simulink model "scalar_training_simulink"  (R2024a)
settings: Solver=FixedStepAuto  StartTime=0.0  StopTime=time(end)  FixedStep=ST  RelTol=1e-3
values from neighbouring files (symbols this model uses):
  c_init = (1/n_nodes)*ones(1, n_nodes)    [scalar_training_init.m]
  delta = 1.2*u_amplitude/(n_nodes/2)    (= 0.072)    [scalar_training_init.m]
  k_a = 0.1    [scalar_training_init.m]
  n_nodes = 50    [scalar_training_init.m]
  ST = 1    [scalar_training_init.m]
settings Model: Creator=gabri  LastModifiedBy=gabri

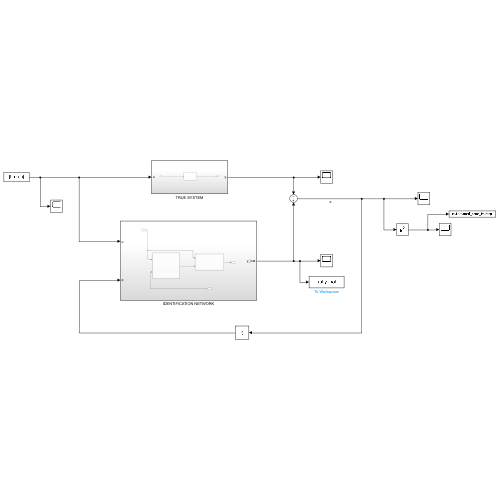
[thumbnail: Simulink's stored preview of the top-level diagram]
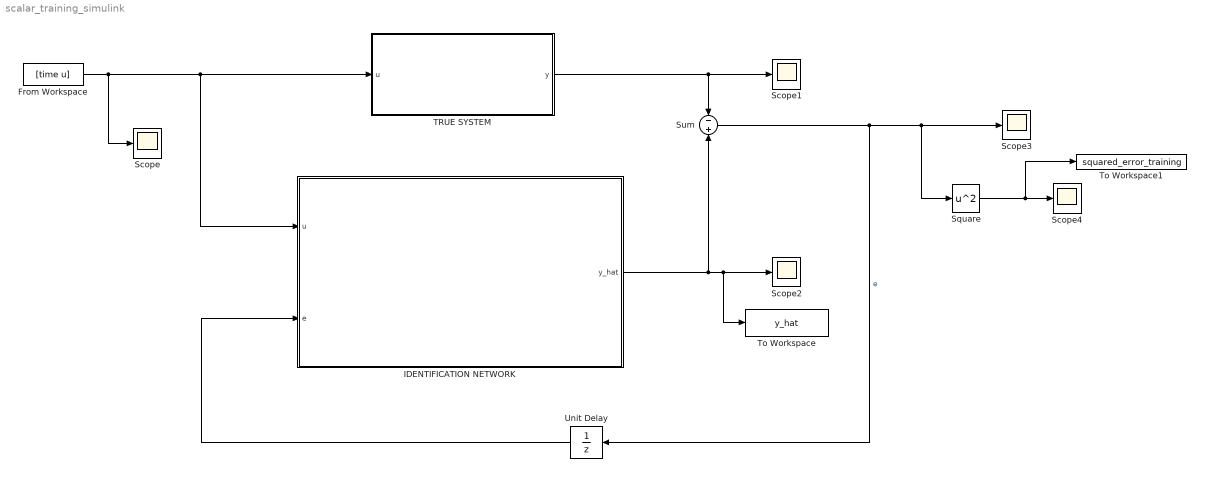
== system scalar_training_simulink ==
  From Workspace : FromWorkspace  VariableName=[time u]  SampleTime=ST
  IDENTIFICATION NETWORK : Subsystem
  Scope{,1..4} (5 alike) : Scope
  Square : Math  Operator=square
  Sum : Sum  Inputs=-|+
  TRUE SYSTEM : Subsystem
  To Workspace : ToWorkspace  VariableName=y_hat  SaveFormat=Timeseries  SampleTime=-1
  To Workspace1 : ToWorkspace  VariableName=squared_error_training  SaveFormat=Timeseries  SampleTime=-1
  Unit Delay : UnitDelay  SampleTime=ST  HasFrameUpgradeWarning=on
  wires:
  From Workspace/1 -> IDENTIFICATION NETWORK/1(u), TRUE SYSTEM/1(u), Scope/1
  TRUE SYSTEM/1(y) -> Sum/1, Scope1/1
  Sum/1 -> Scope3/1, Square/1, Unit Delay/1  "e"
  Square/1 -> To Workspace1/1, Scope4/1
  IDENTIFICATION NETWORK/1(y_hat) -> To Workspace/1, Scope2/1, Sum/2
  Unit Delay/1 -> IDENTIFICATION NETWORK/2(e)

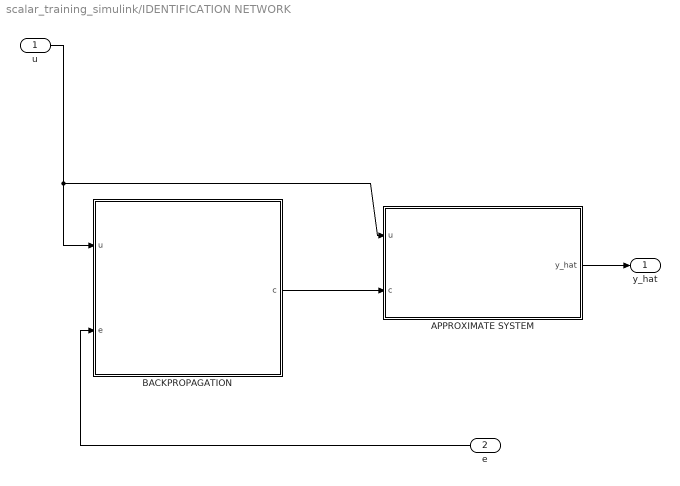
== system scalar_training_simulink/IDENTIFICATION NETWORK ==
  u : Inport
  e : Inport  Port=2
  APPROXIMATE SYSTEM : Subsystem
  BACKPROPAGATION : Subsystem
  y_hat : Outport
  wires:
  BACKPROPAGATION/1(c) -> APPROXIMATE SYSTEM/2(c)
  u/1 -> BACKPROPAGATION/1(u), APPROXIMATE SYSTEM/1(u)
  APPROXIMATE SYSTEM/1(y_hat) -> y_hat/1
  e/1 -> BACKPROPAGATION/2(e)

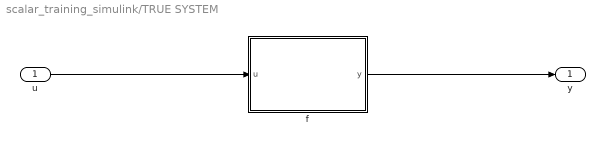
== system scalar_training_simulink/TRUE SYSTEM ==
  u : Inport
  f : MATLAB Function  TreatAsAtomicUnit=on
  y : Outport
  wires:
  u/1 -> f/1(u)
  f/1(y) -> y/1

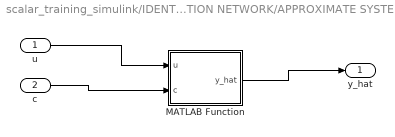
== system scalar_training_simulink/IDENTIFICATION NETWORK/APPROXIMATE SYSTEM ==
  u : Inport
  c : Inport  Port=2
  MATLAB Function : MATLAB Function  TreatAsAtomicUnit=on
  y_hat : Outport
  wires:
  u/1 -> MATLAB Function/1(u)
  MATLAB Function/1(y_hat) -> y_hat/1
  c/1 -> MATLAB Function/2(c)

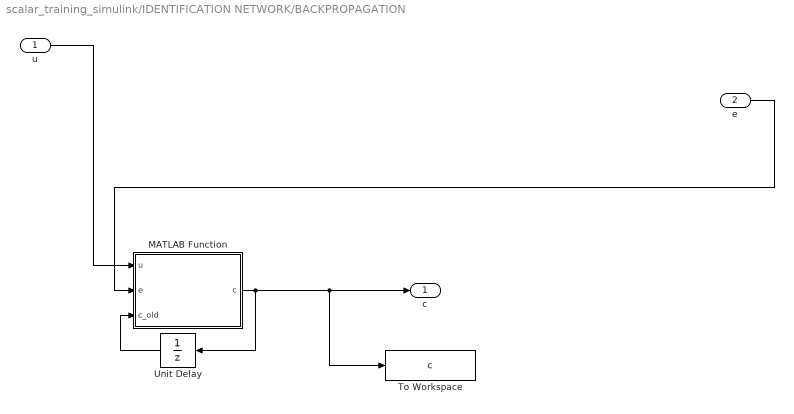
== system scalar_training_simulink/IDENTIFICATION NETWORK/BACKPROPAGATION ==
  u : Inport
  e : Inport  Port=2
  MATLAB Function : MATLAB Function  TreatAsAtomicUnit=on
  To Workspace : ToWorkspace  VariableName=c  SaveFormat=Timeseries  SampleTime=-1
  Unit Delay : UnitDelay  InitialCondition=c_init  SampleTime=ST  HasFrameUpgradeWarning=on
  c : Outport
  wires:
  u/1 -> MATLAB Function/1(u)
  Unit Delay/1 -> MATLAB Function/3(c_old)
  MATLAB Function/1(c) -> To Workspace/1, c/1, Unit Delay/1
  e/1 -> MATLAB Function/2(e)

== matlab function scalar_training_simulink/IDENTIFICATION NETWORK/APPROXIMATE SYSTEM/MATLAB Function ==
  data: u input; y_hat output; c input; delta parameter; n_nodes parameter
function y_hat = f_hat(u, c, delta, n_nodes)

y_hat_temp = 0;

shift = ceil(n_nodes/2);

for i = 1:length(c)
    k = i-shift;
    y_hat_temp = y_hat_temp + c(i)*grf(u, k, delta);
end

y_hat = y_hat_temp;

== matlab function scalar_training_simulink/TRUE SYSTEM/f ==
  data: u input; y output
function y = fcn(u)

y = true_system(u);

== matlab function scalar_training_simulink/IDENTIFICATION NETWORK/BACKPROPAGATION/MATLAB Function ==
  data: u input; e input; c_old input; c output; delta parameter; k_a parameter; n_nodes parameter
function c = c_update(u, e, c_old, delta, k_a, n_nodes)

c_temp = c_old;

shift = ceil(n_nodes/2);

for i = 1:length(c_old)
    k = i-shift;
    c_temp(i) = c_temp(i) - k_a * e * grf(u, k, delta);
end

c = c_temp;
